simulink model "Kalman_Filter_Memory_BlocksETR07"  (R2017b)
settings: Solver=VariableStepAuto  StartTime=0.0  StopTime=10.0  RelTol=1e-3
undefined symbols (not defined in the file or in its folder): s
settings Model: Creator=cspt  LastModifiedBy=cspt
settings SolverCC: AlgebraicLoopSolver=LineSearch

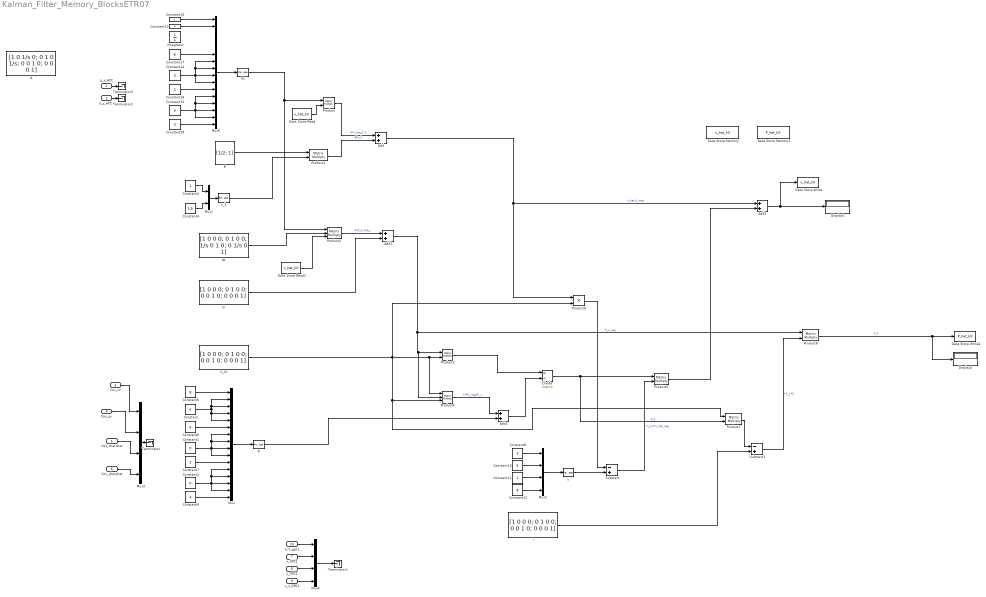
== system Kalman_Filter_Memory_BlocksETR07 ==
  a_x_ACC : Inport
  a_y_ACC : Inport  Port=2
  Cov_xx : Inport  Port=3
  "Cov_yy " : Inport  Port=4
  Cov_xhatxhat : Inport  Port=5
  Cov_yhatyhat : Inport  Port=6
  x_GPS1 : Inport  Port=7
  y_GPS1 : Inport  Port=8
  v_x_GPS1 : Inport  Port=9
  V_Y_gps1 : Inport  Port=10
  A : Constant  Value=[1 0 1/s 0; 0 1 0 1/s; 0 0 1 0; 0 0 0 1]
  Add{,1..3} (4 alike) : Sum
  At : Constant  Value=[1 0 0 0; 0 1 0 0; 1/s 0 1 0; 0 1/s 0 1]
  B : Constant  Value=[1/2; 1]
  C_Ct : Constant  Value=[1 0 0 0; 0 1 0 0; 0 0 1 0; 0 0 0 1]
  Constant{,1..2,13..15} (6 alike) : Constant  Value=0
  Constant10 : Constant  Value=9
  Constant11 : Constant
  Constant12 : Constant  Value=8
  Constant16 : Constant
  Constant17 : Constant  Value=6
  Constant18 : Constant  Value=2
  Constant19 : Constant  Value=3
  Constant3 : Constant
  Constant4 : Constant  Value=1.5
  Constant5 : Constant  Value=8
  Constant6 : Constant  Value=6
  Constant7 : Constant  Value=2
  Constant8 : Constant  Value=3
  Constant9 : Constant  Value=3
  Data Store Memory : DataStoreMemory  DataStoreName=x_hat_k0  ReadBeforeWriteMsg=warning  WriteAfterWriteMsg=warning  WriteAfterReadMsg=warning  ShowAdditionalParam=off
  Data Store Memory1 : DataStoreMemory  DataStoreName=P_hat_k0  ReadBeforeWriteMsg=warning  WriteAfterWriteMsg=warning  WriteAfterReadMsg=warning  ShowAdditionalParam=off
  Data Store Read : DataStoreRead  DataStoreName=x_hat_k0
  Data Store Read1 : DataStoreRead  DataStoreName=x_hat_k0
  Data Store Write : DataStoreWrite  DataStoreName=x_hat_k0
  Data Store Write1 : DataStoreWrite  DataStoreName=P_hat_k0
  Display1 : Display
  Display2 : Display
  Divide : Product  Inputs=*/  Multiplication=Matrix(*)
  I : Constant  Value=[1 0 0 0; 0 1 0 0; 0 0 1 0; 0 0 0 1]
  Integrator : Integrator
  Mux : Mux  Inputs=16
  Mux1 : Mux  Inputs=2
  Mux2 : Mux
  Mux3 : Mux
  Mux4 : Mux
  Mux5 : Mux  Inputs=16
  Product{,1,3,5,7..8} (6 alike) : Product  Multiplication=Matrix(*)
  Product2 : Product  Inputs=3  Multiplication=Matrix(*)
  Product4 : Product  Inputs=3  Multiplication=Matrix(*)
  Product6 : Product
  Q : Constant  Value=[1 0 0 0; 0 1 0 0; 0 0 1 0; 0 0 0 1]
  R : Reshape  OutputDimensionality=Customize  OutputDimensions=[4,4]
  R1 : Reshape  OutputDimensionality=Customize  OutputDimensions=[4,4]
  Subtract : Sum  Inputs=-+
  Subtract1 : Sum  Inputs=-+
  Terminator{,1..3} (4 alike) : Terminator
  u_k : Reshape  OutputDimensionality=Customize  OutputDimensions=[2,1]
  "y " : Reshape  OutputDimensionality=Customize  OutputDimensions=[4,4]
  wires:
  I/1 -> Subtract1/2
  Subtract/1 -> Product5/2  "Y_k-C*x_hat_neg"
  Product8/1 -> Display2/1, Data Store Write1/1  "P_k"
  Constant5/1 -> Mux/1
  At/1 -> Product2/2
  Constant3/1 -> Mux1/1
  Constant/1 -> Mux/5, Mux/4, Mux/3, Mux/2
  Constant4/1 -> Mux1/2
  Product/1 -> Add/1  "A*x_hat_k-1"
  Q/1 -> Add1/2
  Mux1/1 -> u_k/1
  Product2/1 -> Add1/1  "A*P_k-1*A_t"
  Product1/1 -> Add/2  "B*u_k"
  u_k/1 -> Product1/2
  Constant2/1 -> Mux/12, Mux/13, Mux/14, Mux/15
  Constant7/1 -> Mux/11
  Add3/1 -> Display1/1, Data Store Write/1
  Mux/1 -> R/1
  "y "/1 -> Subtract/2
  Product5/1 -> Add3/2
  B/1 -> Product1/1
  Add2/1 -> Divide/2
  Add/1 -> Add3/1, Product6/1  "x_hat_k_neg"
  Subtract1/1 -> Product8/2  "I-K_k*C"
  Mux2/1 -> "y "/1
  Constant9/1 -> Mux/16
  Constant1/1 -> Mux/7, Mux/8, Mux/9, Mux/10
  Constant10/1 -> Mux2/2
  Constant8/1 -> Mux2/1
  Product7/1 -> Subtract1/1
  R1/1 -> Product2/1, Product/1
  Constant11/1 -> Mux2/3
  R/1 -> Add2/2
  Add1/1 -> Product4/2, Product3/1, Product8/1  "P_k_neg"
  C_Ct/1 -> Product6/2, Product4/1, Product3/2, Product4/3, Product7/1
  Product4/1 -> Add2/1  "C*Pk_neg*C_t"
  Divide/1 -> Product7/2, Product5/1  "K_k"
  Constant12/1 -> Mux2/4
  Product6/1 -> Subtract/1
  Product3/1 -> Divide/1
  Constant6/1 -> Mux/6
  Data Store Read/1 -> Product/2
  Data Store Read1/1 -> Product2/3
  Cov_yhatyhat/1 -> Mux3/4
  Cov_xhatxhat/1 -> Mux3/3
  Mux3/1 -> Terminator/1
  "Cov_yy "/1 -> Mux3/2
  Cov_xx/1 -> Mux3/1
  x_GPS1/1 -> Mux4/2
  V_Y_gps1/1 -> Mux4/1
  v_x_GPS1/1 -> Mux4/4
  y_GPS1/1 -> Mux4/3
  Mux4/1 -> Terminator1/1
  a_y_ACC/1 -> Terminator2/1
  a_x_ACC/1 -> Terminator3/1
  Constant16/1 -> Mux5/1
  Mux5/1 -> R1/1
  Constant19/1 -> Mux5/16
  Constant13/1 -> Mux5/2
  Constant15/1 -> Mux5/12, Mux5/13, Mux5/14, Mux5/15
  Constant18/1 -> Mux5/11
  Constant17/1 -> Mux5/6
  Constant14/1 -> Mux5/7, Mux5/8, Mux5/9, Mux5/10
